simulink model "Estimator_Simulink_J2"  (R2018b)
settings: Solver=VariableStepAuto  StartTime=0.0  StopTime=90000  RelTol=1e-3
InitFcn:
  | load('Sim_Truth_SecondOrder_Corrected5.mat')
values from neighbouring files (symbols this model uses):
  A = [-1/(Rc*Cc) 0; 0 0]    [BatteryModel_1stOrder_Youla.m]    (also in Estimator_Simulink_driver.m = [1 0 ; 0 (1-(dt/(Rc*Cc)))]; battery_equivalent_circuit_model_KF.m = 1)
  B = [1/Cc; -1/Cbat]    [BatteryModel_1stOrder_Youla.m]    (also in Estimator_Simulink_driver.m = [-(dt/Cbat) ; (dt/Cc)]; battery_equivalent_circuit_model_KF.m = -5.55555555556e-06)
  C = [-1 alpha]    [BatteryModel_1stOrder_Youla.m]    (also in Estimator_Simulink_driver.m = [alpha -1]; battery_equivalent_circuit_model_KF.m = 0.65)
  D = -R0    (= -0.1)    [BatteryModel_1stOrder_Youla.m]    (also in Estimator_Simulink_driver.m = [-R0]; battery_equivalent_circuit_model_KF.m = -0.01)
  Vocv0 = 3.435    [BatteryModel_1stOrder_Youla.m]    (also in Estimator_Simulink_driver.m; battery_equivalent_circuit_model_KF.m)
undefined symbols (not defined in the file or in its folder): den, num
libraries: dspsrcs4 x3, dspstat3 x2
settings Model: Creator=Indiana  LastModifiedBy=felip

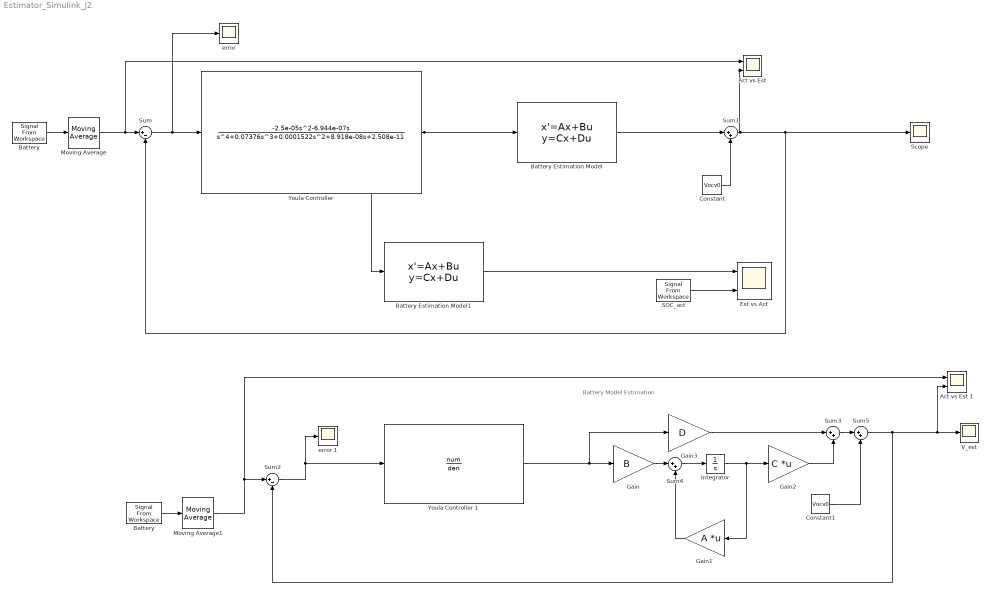
== system Estimator_Simulink_J2 ==
  note: Battery Model Estimation
  "Act vs Est " : Scope  NumInputPorts=2
  Act vs Est 1 : Scope  NumInputPorts=2
  Battery : dspsrcs4/Signal From Workspace  X=V  Ts=1  nsamps=1  OutputAfterFinalValue=Setting to zero  ignoreOrWarnInputAndFrameLengths=off  OutputFrames=off
  "Battery " : dspsrcs4/Signal From Workspace  X=V  Ts=1  nsamps=1  OutputAfterFinalValue=Setting to zero  ignoreOrWarnInputAndFrameLengths=off  OutputFrames=off
  Battery Estimation Model : StateSpace  A=A  B=B  C=C  D=D  InitialCondition=[0; 1]
  Battery Estimation Model1 : StateSpace  A=A  B=B  C=[0,1]  D=0  InitialCondition=[0; 1]
  Constant : Constant  Value=Vocv0
  Constant1 : Constant  Value=Vocv0
  "Est vs Act " : Scope  NumInputPorts=2
  Gain : Gain  Gain=B
  Gain1 : Gain  Gain=A  Multiplication=Matrix(K*u)
  Gain2 : Gain  Gain=C  Multiplication=Matrix(K*u)
  Gain3 : Gain  Gain=D
  Integrator : Integrator
  Moving Average : dspstat3/Moving Average  Method=Sliding window  ForgettingFactorPort=off  SpecifyWindowLength=on  WindowLength=10  ForgettingFactor=0.9  SimulateUsing=Code generation
  Moving Average1 : dspstat3/Moving Average  Method=Sliding window  ForgettingFactorPort=off  SpecifyWindowLength=on  WindowLength=10  ForgettingFactor=0.9  SimulateUsing=Code generation
  "SOC_act " : dspsrcs4/Signal From Workspace  X=SOC_act  Ts=1  nsamps=1  OutputAfterFinalValue=Setting to zero  ignoreOrWarnInputAndFrameLengths=off  OutputFrames=off
  Scope : Scope
  Sum : Sum  Inputs=|+-
  Sum{1,3..5} (4 alike) : Sum  Inputs=|++
  Sum2 : Sum  Inputs=|+-
  "V_est " : Scope
  "Youla Controller " : TransferFcn  Numerator=[-2.5e-05 -6.944e-07 0]  Denominator=[1 0.07376 0.0001522 8.918e-08 2.508e-11]
  Youla Controller 1 : TransferFcn  Numerator=num  Denominator=den
  "error " : Scope
  error 1 : Scope
  wires:
  "Battery "/1 -> Moving Average/1
  "Youla Controller "/1 -> Battery Estimation Model/1, Battery Estimation Model1/1
  Battery Estimation Model/1 -> Sum1/1
  Sum/1 -> "error "/1, "Youla Controller "/1
  Moving Average/1 -> Sum/1, "Act vs Est "/1
  Battery Estimation Model1/1 -> "Est vs Act "/1
  "SOC_act "/1 -> "Est vs Act "/2
  Constant/1 -> Sum1/2
  Sum1/1 -> Sum/2, Scope/1, "Act vs Est "/2
  Moving Average1/1 -> Act vs Est 1/1, Sum2/1
  Battery/1 -> Moving Average1/1
  Sum2/1 -> error 1/1, Youla Controller 1/1
  Sum5/1 -> "V_est "/1, Act vs Est 1/2, Sum2/2
  Constant1/1 -> Sum5/2
  Youla Controller 1/1 -> Gain3/1, Gain/1
  Sum3/1 -> Sum5/1
  Gain3/1 -> Sum3/1
  Gain2/1 -> Sum3/2
  Gain1/1 -> Sum4/2
  Sum4/1 -> Integrator/1
  Integrator/1 -> Gain1/1, Gain2/1
  Gain/1 -> Sum4/1
